simulink model "LAB2_Mass_spring_dumper"  (R2022b)
settings: Solver=FixedStepAuto  StartTime=to  StopTime=tf  FixedStep=0.1  RelTol=1e-3
values from neighbouring files (symbols this model uses):
  b = 5    [LAB_02.m]
  k = 6    [LAB_02.m]
  m = 2    [LAB_02.m]
  omega = 0.5    [LAB_02.m]
  v0 = [3.021; 24.139; 10.964]    [LAB_02.m]
  x0 = 1    [LAB_02.m]
settings Model: Creator=ludov  LastModifiedBy=ludov

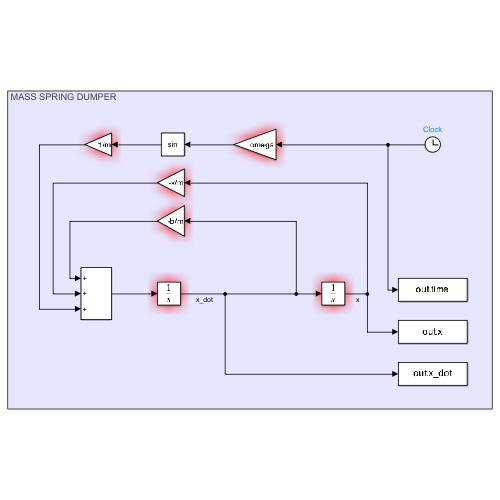
[thumbnail: Simulink's stored preview of the top-level diagram]
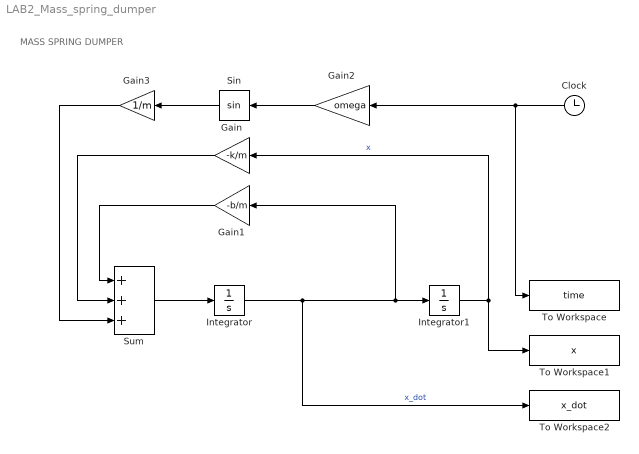
== system LAB2_Mass_spring_dumper ==
  note: MASS SPRING DUMPER
  Clock : Clock
  Gain : Gain  Gain=-k/m
  Gain1 : Gain  Gain=-b/m
  Gain2 : Gain  Gain=omega
  Gain3 : Gain  Gain=1/m
  Integrator : Integrator  InitialCondition=v0
  Integrator1 : Integrator  InitialCondition=x0
  Sin : Trigonometry
  Sum : Sum  Inputs=+++
  To Workspace : ToWorkspace  VariableName=time  SaveFormat=Timeseries  SampleTime=-1
  To Workspace1 : ToWorkspace  VariableName=x  SaveFormat=Timeseries  SampleTime=-1
  To Workspace2 : ToWorkspace  VariableName=x_dot  SaveFormat=Timeseries  SampleTime=-1
  wires:
  Integrator/1 -> Integrator1/1, Gain1/1, To Workspace2/1  "x_dot"
  Integrator1/1 -> To Workspace1/1, Gain/1  "x"
  Gain1/1 -> Sum/1
  Gain/1 -> Sum/2
  Clock/1 -> To Workspace/1, Gain2/1
  Gain2/1 -> Sin/1
  Sin/1 -> Gain3/1
  Sum/1 -> Integrator/1
  Gain3/1 -> Sum/3
